simulink library "beb"  (Simulink 8.1)
settings: Solver=ode1  StartTime=0.0  StopTime=Inf  FixedStep=0.001  RelTol=1e-3
PostLoadFcn:
  | , if any(exist('dsrtsu_mdlpostloadfcn', 'file') == [2, 3, 6]), try dsrtsu_mdlpostloadfcn('Execute', bdroot); catch fprintf('Error in PostLoadFcn (dsrtsu_mdlpostloadfcn) for model "%s":\n %s\n', bdroot, lasterr); end, end,
undefined symbols (not defined in the file or in its folder): FALSE, KAEB_HoldModeLimitSpeed_kph, KAEB_WarnLightsDecel_mps2, KAEB_WarnLightSpeedThresh_kph, ZERO_FLOAT
settings Model: DSRTSU_INTERNAL_RTI_VER=450  DSRTSU_INTERNAL_RTI_TYPE=rti1401  RTICANMMDATA=struct('GeneralSetupData',struct('modelroot','D:\PROJECTS\HAITEC\TAIWAN_HAITEC_SVN\trunk\AdasDragon\software\sw_development\arch\app\aeb','generalsettings',struct('filesettings',struct('destfolder',struct('Name','RTICANMM_FILES','Check',1),'buildfolder',struct('Name','.','Check',1),'AbsDestfolder',struct('Name','D:\PROJECTS\HAITEC\TAIWAN_HAITEC_SVN\trunk\AdasDragon\software\sw_development\arch\app\aeb\RTICANMM_FILES'),'AbsBuildfolder',struct('Name','D:\PROJECTS\HAITEC\TAIWAN_HAITEC_SVN\trunk\AdasDragon\software\sw_development\arch\app\aeb'))),'options',struct('addpaths',1,'rmpaths',1,'addtrcexclusion',logical(1),'cannavigator',struct('checkmonitoring',0),'show_usrtrc',0,'use_usrtrc',0),'advanced',struct('options',[1 1 1 1 1 1 1 1 1 1 1 1 1 1 1 1 1 1 1 1 1 1 1 1 1 1 1 1 1 1 1 1 1 1 1 1 1 1 1 1 1 1 1 1 1 1 1 1 1 1 1 1 1 1 1 1 1 1 1 1 1 1 1 1 1 1 1 1 1 1 1 1 1 1 1 1 1 1 1 1 1 1 1 1 1 1 1 1 1 1 1 1 1 1 1 1 1 1 1 1]),'MPSetup',{{}},'modelname','beb','block','beb'))  DSRTSU_INTERNAL_RTIFPGA=40  Creator=tescamilla  LastModifiedBy=tescamilla

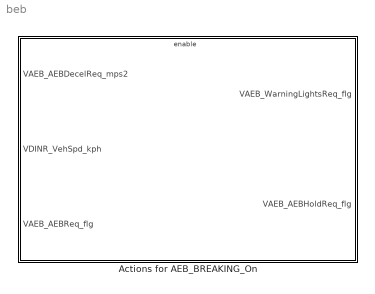
== system beb ==
  Actions for AEB_BREAKING_On : Subsystem  TreatAsAtomicUnit=on

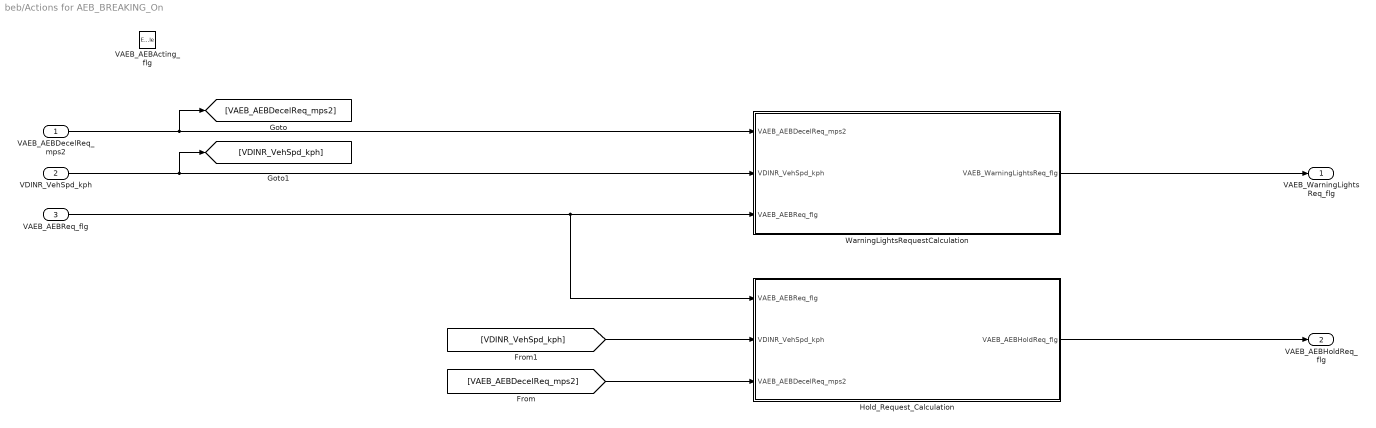
== system beb/Actions for AEB_BREAKING_On ==
  VAEB_AEBDecelReq_mps2 : Inport
  VDINR_VehSpd_kph : Inport  Port=2
  VAEB_AEBReq_flg : Inport  Port=3
  VAEB_AEBActing_flg : EnablePort  StatesWhenEnabling=reset
      settings: AttributesFormatString=State=%<StatesWhenEnabling>
  Hold_Request_Calculation : Subsystem
  WarningLightsRequestCalculation : Subsystem
  VAEB_WarningLightsReq_flg : Outport  OutputWhenDisabled=reset  InitialOutput=FALSE
  VAEB_AEBHoldReq_flg : Outport  Port=2  OutputWhenDisabled=reset  InitialOutput=FALSE
  wires:
  VDINR_VehSpd_kph/1 -> [VDINR_VehSpd_kph], WarningLightsRequestCalculation/2(VDINR_VehSpd_kph)
  VAEB_AEBDecelReq_mps2/1 -> WarningLightsRequestCalculation/1(VAEB_AEBDecelReq_mps2), [VAEB_AEBDecelReq_mps2]
  [VAEB_AEBDecelReq_mps2] -> Hold_Request_Calculation/3(VAEB_AEBDecelReq_mps2)
  [VDINR_VehSpd_kph] -> Hold_Request_Calculation/2(VDINR_VehSpd_kph)
  VAEB_AEBReq_flg/1 -> Hold_Request_Calculation/1(VAEB_AEBReq_flg), WarningLightsRequestCalculation/3(VAEB_AEBReq_flg)
  WarningLightsRequestCalculation/1(VAEB_WarningLightsReq_flg) -> VAEB_WarningLightsReq_flg/1
  Hold_Request_Calculation/1(VAEB_AEBHoldReq_flg) -> VAEB_AEBHoldReq_flg/1

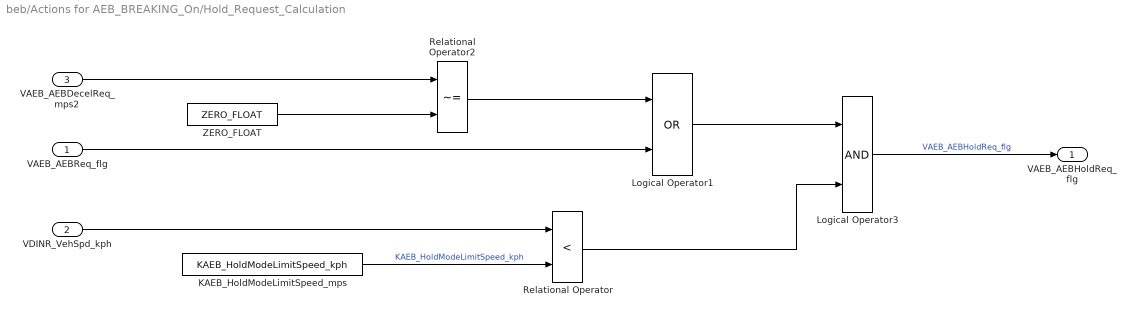
== system beb/Actions for AEB_BREAKING_On/Hold_Request_Calculation ==
  VAEB_AEBReq_flg : Inport
  VDINR_VehSpd_kph : Inport  Port=2
  VAEB_AEBDecelReq_mps2 : Inport  Port=3
  KAEB_HoldModeLimitSpeed_mps : Constant  Value=KAEB_HoldModeLimitSpeed_kph  OutDataTypeStr=single
  Logical Operator1 : Logic  Operator=OR  AllPortsSameDT=off  OutDataTypeStr=boolean
  Logical Operator3 : Logic  AllPortsSameDT=off  OutDataTypeStr=boolean
  Relational Operator : RelationalOperator  Operator=<  OutDataTypeStr=boolean
  Relational Operator2 : RelationalOperator  Operator=~=  OutDataTypeStr=boolean
  ZERO_FLOAT : Constant  Value=ZERO_FLOAT  OutDataTypeStr=single
  VAEB_AEBHoldReq_flg : Outport
  wires:
  Relational Operator2/1 -> Logical Operator1/1
  ZERO_FLOAT/1 -> Relational Operator2/2
  VAEB_AEBDecelReq_mps2/1 -> Relational Operator2/1
  Logical Operator3/1 -> VAEB_AEBHoldReq_flg/1  "VAEB_AEBHoldReq_flg"
  VAEB_AEBReq_flg/1 -> Logical Operator1/2
  Logical Operator1/1 -> Logical Operator3/1
  KAEB_HoldModeLimitSpeed_mps/1 -> Relational Operator/2  "KAEB_HoldModeLimitSpeed_kph"
  VDINR_VehSpd_kph/1 -> Relational Operator/1
  Relational Operator/1 -> Logical Operator3/2

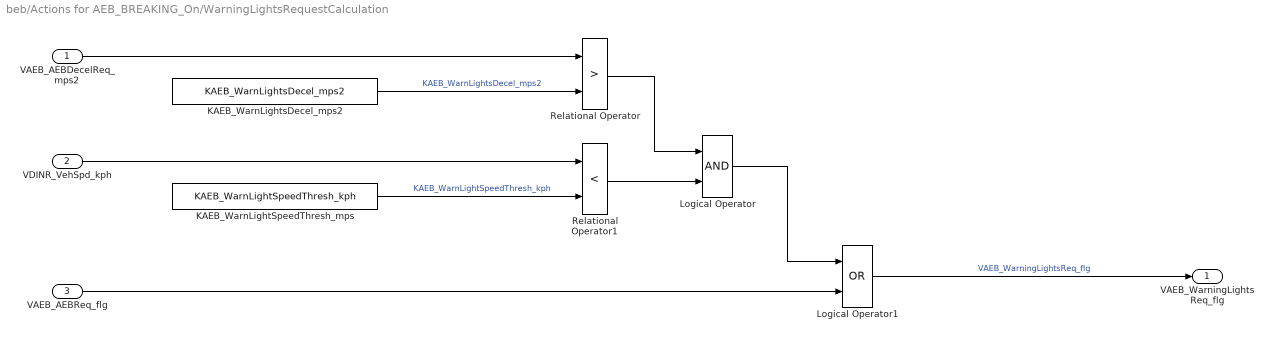
== system beb/Actions for AEB_BREAKING_On/WarningLightsRequestCalculation ==
  VAEB_AEBDecelReq_mps2 : Inport
  VDINR_VehSpd_kph : Inport  Port=2
  VAEB_AEBReq_flg : Inport  Port=3
  KAEB_WarnLightSpeedThresh_mps : Constant  Value=KAEB_WarnLightSpeedThresh_kph  OutDataTypeStr=single
  KAEB_WarnLightsDecel_mps2 : Constant  Value=KAEB_WarnLightsDecel_mps2  OutDataTypeStr=single
  Logical Operator : Logic  AllPortsSameDT=off  OutDataTypeStr=boolean
  Logical Operator1 : Logic  Operator=OR  AllPortsSameDT=off  OutDataTypeStr=boolean
  Relational Operator : RelationalOperator  Operator=>  OutDataTypeStr=boolean
  Relational Operator1 : RelationalOperator  Operator=<  OutDataTypeStr=boolean
  VAEB_WarningLightsReq_flg : Outport
  wires:
  KAEB_WarnLightsDecel_mps2/1 -> Relational Operator/2  "KAEB_WarnLightsDecel_mps2"
  VAEB_AEBDecelReq_mps2/1 -> Relational Operator/1
  KAEB_WarnLightSpeedThresh_mps/1 -> Relational Operator1/2  "KAEB_WarnLightSpeedThresh_kph"
  VDINR_VehSpd_kph/1 -> Relational Operator1/1
  Logical Operator1/1 -> VAEB_WarningLightsReq_flg/1  "VAEB_WarningLightsReq_flg"
  Relational Operator/1 -> Logical Operator/1
  Relational Operator1/1 -> Logical Operator/2
  Logical Operator/1 -> Logical Operator1/1
  VAEB_AEBReq_flg/1 -> Logical Operator1/2
